simulink library "winch000_cl"  (R2018b)
settings: Solver=VariableStepAuto  StartTime=0.0  StopTime=10.0  RelTol=1e-3
undefined symbols (not defined in the file): wnch
libraries: firstOrderFilter_ul x1
settings Model: Creator=mcobb  LastModifiedBy=mcobb

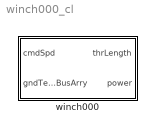
== system winch000_cl ==
  winch000 : Subsystem  VariantControl=VSS_winch_winch000

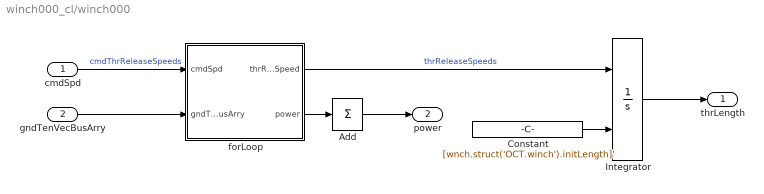
== system winch000_cl/winch000 ==
  cmdSpd : Inport
  gndTenVecBusArry : Inport  Port=2
  Add : Sum  Inputs=+
  Constant : Constant  Value=[wnch.struct('OCT.winch').initLength]'  VectorParams1D=off
  Integrator : Integrator  InitialConditionSource=external
  forLoop : Subsystem  mask{wnch=wnch.struct('OCT.winch')}
      mask prompts: wnch "Winch Structure"
  thrLength : Outport
  power : Outport  Port=2
  wires:
  gndTenVecBusArry/1 -> forLoop/2(gndTenVecBusArry)
  forLoop/2(power) -> Add/1
  forLoop/1(thrReleaseSpeed) -> Integrator/1  "thrReleaseSpeeds"
  Add/1 -> power/1
  Constant/1 -> Integrator/2
  Integrator/1 -> thrLength/1
  cmdSpd/1 -> forLoop/1(cmdSpd)  "cmdThrReleaseSpeeds"

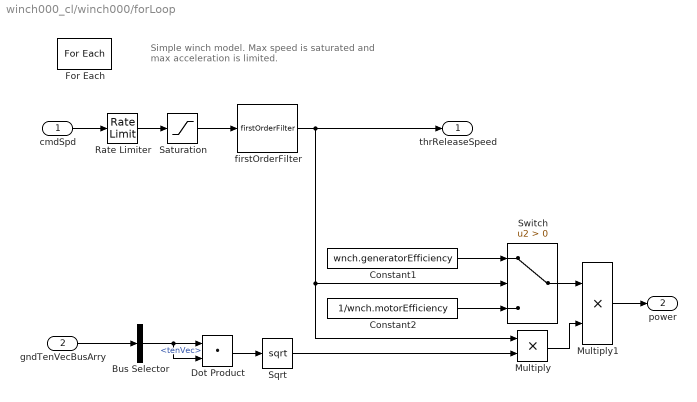
== system winch000_cl/winch000/forLoop ==
  note: Simple winch model.  Max speed is saturated
      | and max acceleration is limited.
  cmdSpd : Inport  Partition=on  PartitionDimension=1  PartitionWidth=1  PartitionOffset=0
  gndTenVecBusArry : Inport  Port=2  Partition=on  PartitionDimension=1  PartitionWidth=1  PartitionOffset=0
  Bus Selector : BusSelector  OutputSignals=tenVec
  Constant1 : Constant  Value=wnch.generatorEfficiency
  Constant2 : Constant  Value=1/wnch.motorEfficiency
  Dot Product : DotProduct  InputSameDT=on  OutDataTypeStr=Inherit: Inherit via internal rule
  For Each : ForEach  DisableCoverage=on  IterateSubsysMaskParameter=on  SubsysMaskParameterIterationDimension=2  IndexMode=One-based
  Multiply : Product
  Multiply1 : Product
  Rate Limiter : RateLimiter  RisingSlewLimit=wnch.maxAccel  FallingSlewLimit=-wnch.maxAccel  SampleTimeMode=inherited
  Saturation : Saturate  UpperLimit=wnch.maxSpeed  LowerLimit=-wnch.maxSpeed  LinearizeAsGain=off
  Sqrt : Sqrt  SaturateOnIntegerOverflow=on
  Switch : Switch  Criteria=u2 > Threshold
  firstOrderFilter : firstOrderFilter_ul/firstOrderFilter  tau=wnch.timeConst  ic=0
  thrReleaseSpeed : Outport  ConcatenationDimension=1
  power : Outport  Port=2  ConcatenationDimension=1
  wires:
  Multiply/1 -> Multiply1/2
  Sqrt/1 -> Multiply/2
  Dot Product/1 -> Sqrt/1
  Bus Selector/1 -> Dot Product/1, Dot Product/2  "<tenVec>"
  gndTenVecBusArry/1 -> Bus Selector/1
  Saturation/1 -> firstOrderFilter/1
  Rate Limiter/1 -> Saturation/1
  firstOrderFilter/1 -> thrReleaseSpeed/1, Switch/2, Multiply/1
  cmdSpd/1 -> Rate Limiter/1
  Switch/1 -> Multiply1/1
  Constant1/1 -> Switch/1
  Constant2/1 -> Switch/3
  Multiply1/1 -> power/1
